simulink model "multiModeQuad_ROS"  (R2021b)
settings: Solver=FixedStepAuto  StartTime=0.0  StopTime=Inf  FixedStep=0.002  RelTol=1e-3
model workspace (MAT data in the model file):
  armLength = 0.12
  deltaT = 0.0019
  motorLength = 0.02
  servoLength = 0.03
undefined symbols (not defined in the file): AngularVelocity, Header, LinearAcceleration, Orientation, Pose
libraries: robotlib x12, slpidlib x7, sharedtransform x2, shared6dof x1
settings Model: Creator=hexia  LastModifiedBy=jack
settings OptimizationCC: EnhancedBackFolding=on  PassReuseOutputArgsAs=Individual arguments  ZeroExternalMemoryAtStartup=off  ZeroInternalMemoryAtStartup=off  MaxStackSize=64  OptimizeBlockOrder=speed  DifferentSizesBufferReuse=on  OptimizationCustomize=off  EfficientTunableParamExpr=on
settings DebuggingCC: ParameterTunabilityLossMsg=error
settings HardwareCC: ProdBitPerPointer=32  ProdBitPerSizeT=32  ProdBitPerPtrDiffT=32  ProdLargestAtomicFloat=None  ProdIntDivRoundTo=Undefined  ProdEndianess=Unspecified  ProdWordSize=32  ProdHWDeviceType=Generic->Unspecified (assume 32-bit Generic)
settings SFSimCC: MATLABDynamicMemAlloc=off
settings RTWCC: Description=Embedded Coder  SystemTargetFile=ert.tlc  HardwareBoard=Robot Operating System (ROS)  TLCOptions="-aInlineSetEventsForThisBaseRateFcn=TLC_FALSE -aSuppressMultiTaskScheduler=TLC_FALSE  -aRateBasedStepFcn=0"  TemplateMakefile=ert_default_tmf  Toolchain=Catkin  TargetLang=C++
settings CodeAppCC: ForceParamTrailComments=on  IgnoreCustomStorageClasses=off  OperatorAnnotations=on  SimulinkDataObjDesc=on  SFDataObjDesc=on  InsertBlockDesc=on
settings ERTTargetCC: SupportContinuousTime=on  SupportVariableSizeSignals=on

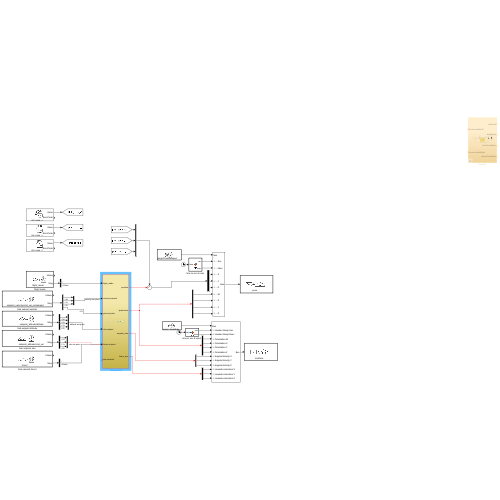
[thumbnail: Simulink's stored preview of the top-level diagram]
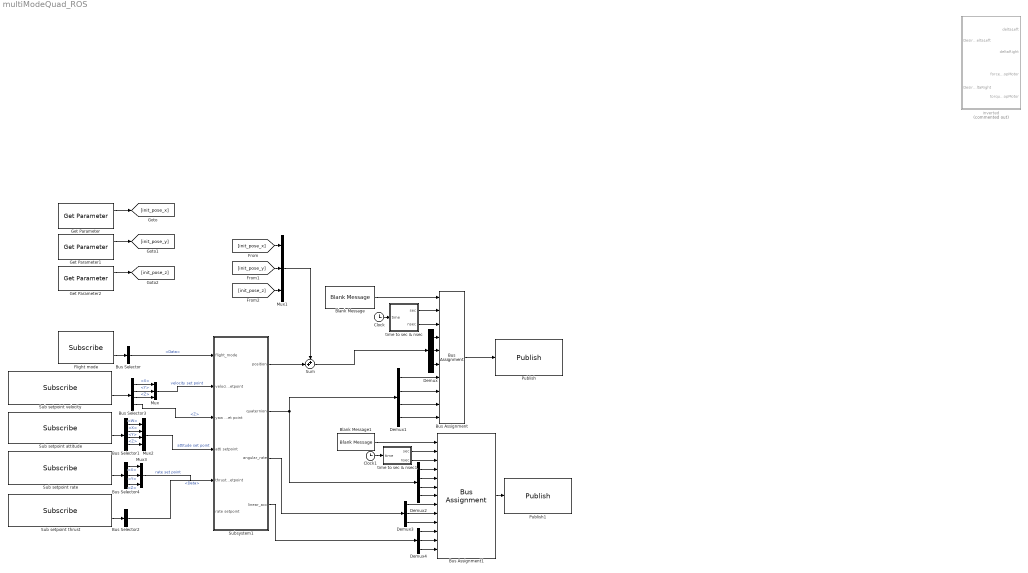
== system multiModeQuad_ROS ==
  Blank Message : robotlib/Blank Message  messageClass=Message  entityType=geometry_msgs/PoseStamped  messageType=geometry_msgs/PoseStamped  SampleTime=inf  legacyBusStruct=off
  Blank Message1 : robotlib/Blank Message  messageClass=Message  entityType=sensor_msgs/Imu  messageType=sensor_msgs/Imu  SampleTime=inf  legacyBusStruct=off
  Bus Assignment : BusAssignment  AssignedSignals=Header.Stamp.Sec,Header.Stamp.Nsec,Pose.Position.X,Pose.Position.Y,Pose.Position.Z,Pose.Orientation.W,Pose.Orientation.X,Pose.Orientation.Y,Pose.Orientation.Z
  Bus Assignment1 : BusAssignment  AssignedSignals=Header.Stamp.Sec,Header.Stamp.Nsec,Orientation.W,Orientation.X,Orientation.Y,Orientation.Z,AngularVelocity.X,AngularVelocity.Y,AngularVelocity.Z,LinearAcceleration.X,LinearAcceleration.Y,LinearAcceleration.Z
  Bus Selector : BusSelector  OutputSignals=Data
  Bus Selector1 : BusSelector  OutputSignals=Pose.Orientation.W,Pose.Orientation.X,Pose.Orientation.Y,Pose.Orientation.Z
  Bus Selector2 : BusSelector  OutputSignals=Data
  Bus Selector3 : BusSelector  OutputSignals=Linear.X,Linear.Y,Linear.Z,Angular.Z
  Bus Selector4 : BusSelector  OutputSignals=Twist.Angular.X,Twist.Angular.Y,Twist.Angular.Z
  Clock : Clock
  Clock1 : Clock
  Demux : Demux  Outputs=3
  Demux1 : Demux
  Demux2 : Demux
  Demux3 : Demux  Outputs=3
  Demux4 : Demux  Outputs=3
  Flight mode : robotlib/Subscribe  topicSource=Specify your own  topic=flight_mode  messageType=std_msgs/Int16  SampleTime=-1  legacyBusStruct=off  messageQueueLength=51
  Get Parameter : robotlib/Get Parameter  ParameterSource=Specify your own  ParameterName=init_pose_x  ParameterType=double  ParameterMaxArrayLength=16  ParameterInitialValue=0.0  SampleTime=-1  ShowErrorCodeOutput=on  ModelName=multiModeQuad_ROS  BlockId=ParamGet_multiModeQuad_ROS_459
      settings: SourceProductBaseCode=RR
  Get Parameter1 : robotlib/Get Parameter  ParameterSource=Specify your own  ParameterName=init_pose_y  ParameterType=double  ParameterMaxArrayLength=16  ParameterInitialValue=0.0  SampleTime=-1  ShowErrorCodeOutput=on  ModelName=multiModeQuad_ROS  BlockId=ParamGet_multiModeQuad_ROS_460
      settings: SourceProductBaseCode=RR
  Get Parameter2 : robotlib/Get Parameter  ParameterSource=Specify your own  ParameterName=init_pose_z  ParameterType=double  ParameterMaxArrayLength=16  ParameterInitialValue=0.0  SampleTime=-1  ShowErrorCodeOutput=on  ModelName=multiModeQuad_ROS  BlockId=ParamGet_multiModeQuad_ROS_461
      settings: SourceProductBaseCode=RR
  Mux : Mux  Inputs=3
  Mux1 : Mux  Inputs=3
  Mux2 : Mux
  Mux3 : Mux  Inputs=3
  Publish : robotlib/Publish  topicSource=Specify your own  topic=pose  messageType=geometry_msgs/PoseStamped  legacyBusStruct=off  messageQueueLength=1
  Publish1 : robotlib/Publish  topicSource=Specify your own  topic=imuData  messageType=sensor_msgs/Imu  legacyBusStruct=off  messageQueueLength=1
  Sub setpoint attitude : robotlib/Subscribe  topicSource=Specify your own  topic=setpoint_attitude/attitude  messageType=geometry_msgs/PoseStamped  SampleTime=-1  legacyBusStruct=off  messageQueueLength=51
  Sub setpoint rate : robotlib/Subscribe  topicSource=Specify your own  topic=setpoint_attitude/cmd_vel  messageType=geometry_msgs/TwistStamped  SampleTime=-1  legacyBusStruct=off  messageQueueLength=51
  Sub setpoint thrust : robotlib/Subscribe  topicSource=Specify your own  topic=thrust  messageType=std_msgs/Float32  SampleTime=-1  legacyBusStruct=off  messageQueueLength=51
  Sub setpoint velocity : robotlib/Subscribe  topicSource=Specify your own  topic=setpoint_velocity/cmd_vel_unstamped  messageType=geometry_msgs/Twist  SampleTime=-1  legacyBusStruct=off  messageQueueLength=51
  Subsystem1 : Subsystem
  Sum : Sum  Inputs=++|
  inverted : Subsystem  Commented=on
  time to sec & nsec : MATLAB Function  TreatAsAtomicUnit=on
  time to sec & nsec1 : MATLAB Function  TreatAsAtomicUnit=on
  wires:
  Mux/1 -> Subsystem1/2(velocity setpoint)  "velocity set point"
  Bus Selector3/4 -> Subsystem1/3(yaw set point)  "<Z>"
  Sub setpoint velocity/2 -> Bus Selector3/1
  Bus Selector3/3 -> Mux/3  "<Z>"
  Bus Selector3/1 -> Mux/1  "<X>"
  Bus Selector3/2 -> Mux/2  "<Y>"
  Blank Message/1 -> Bus Assignment/1
  Bus Assignment/1 -> Publish/1
  Clock/1 -> time to sec & nsec/1(time)
  time to sec & nsec/1(sec) -> Bus Assignment/2
  time to sec & nsec/2(nsec) -> Bus Assignment/3
  Demux/1 -> Bus Assignment/4
  Demux/2 -> Bus Assignment/5
  Demux/3 -> Bus Assignment/6
  Sum/1 -> Demux/1
  Demux1/1 -> Bus Assignment/7
  Demux1/2 -> Bus Assignment/8
  Demux1/3 -> Bus Assignment/9
  Demux1/4 -> Bus Assignment/10
  Get Parameter/1 -> [init_pose_x]
  Get Parameter1/1 -> [init_pose_y]
  Get Parameter2/1 -> [init_pose_z]
  Subsystem1/1(position) -> Sum/2
  Mux1/1 -> Sum/1
  [init_pose_x] -> Mux1/1
  [init_pose_y] -> Mux1/2
  [init_pose_z] -> Mux1/3
  Flight mode/2 -> Bus Selector/1
  Bus Selector/1 -> Subsystem1/1(flight_mode)  "<Data>"
  Bus Assignment1/1 -> Publish1/1
  Blank Message1/1 -> Bus Assignment1/1
  Demux2/2 -> Bus Assignment1/5
  Demux2/4 -> Bus Assignment1/7
  Demux2/1 -> Bus Assignment1/4
  Demux2/3 -> Bus Assignment1/6
  Subsystem1/2(quaternion) -> Demux1/1, Demux2/1
  Demux3/1 -> Bus Assignment1/8
  Demux3/2 -> Bus Assignment1/9
  Demux3/3 -> Bus Assignment1/10
  Subsystem1/3(angular_rate) -> Demux3/1
  Demux4/1 -> Bus Assignment1/11
  Demux4/2 -> Bus Assignment1/12
  Subsystem1/4(linear_acc) -> Demux4/1
  Demux4/3 -> Bus Assignment1/13
  Clock1/1 -> time to sec & nsec1/1(time)
  time to sec & nsec1/1(sec) -> Bus Assignment1/2
  time to sec & nsec1/2(nsec) -> Bus Assignment1/3
  Sub setpoint attitude/2 -> Bus Selector1/1
  Bus Selector1/1 -> Mux2/1  "<W>"
  Bus Selector1/2 -> Mux2/2  "<X>"
  Bus Selector1/3 -> Mux2/3  "<Y>"
  Bus Selector1/4 -> Mux2/4  "<Z>"
  Mux2/1 -> Subsystem1/4(atti setpoint)  "attitude set point"
  Sub setpoint thrust/2 -> Bus Selector2/1
  Bus Selector2/1 -> Subsystem1/5(thrust setpoint)  "<Data>"
  Sub setpoint rate/2 -> Bus Selector4/1
  Bus Selector4/1 -> Mux3/1  "<X>"
  Bus Selector4/2 -> Mux3/2  "<Y>"
  Bus Selector4/3 -> Mux3/3  "<Z>"
  Mux3/1 -> ?  "rate set point"

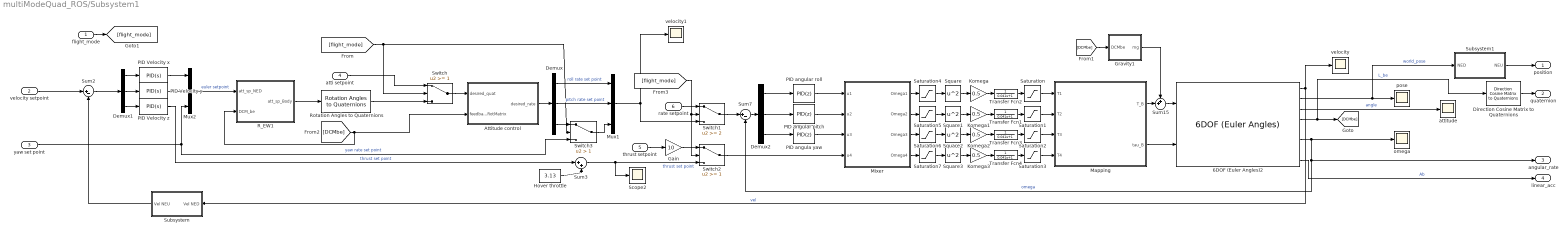
== system multiModeQuad_ROS/Subsystem1 ==
  flight_mode : Inport
  velocity setpoint : Inport  Port=2
  yaw set point : Inport  Port=3
  atti setpoint : Inport  Port=4
  thrust setpoint : Inport  Port=5
  rate setpoint : Inport  Port=6
  6DOF (Euler Angles)2 : shared6dof/6DOF (Euler Angles)  units=Metric (MKS)  mtype=Fixed  rep=Euler Angles  xme_0=[0 0 0]  Vm_0=[0 0 0]  eul_0=[0 0 0]  pm_0=[0 0 0]  mass_0=2  mass_e=0.5  mass_f=2.0  inertia=[0.015 0 0;0 0.015 0; 0 0 0.03]  inertia_e=eye(3)  inertia_f=2*eye(3)  k_quat=1.0  vre_flag=on  abi_flag=off  aMode=aMode  xme_statename=''  Vm_statename=''  eul_statename=''  quat_statename=''  pm_statename=''  mass_statename=''
      settings: SourceProductBaseCode=AE,PW,DR,MT,UV,VE
  Attitude control : MATLAB Function  TreatAsAtomicUnit=on
  Demux : Demux  Outputs=3
  Demux1 : Demux  Outputs=3
  Demux2 : Demux  Outputs=3
  Direction Cosine Matrix to Quaternions : sharedtransform/Direction Cosine Matrix  to Quaternions  aMode=0  action=None  tolerance=eps(2)
      settings: SourceProductBaseCode=AE,PW,DR,MT,UV,VE
  Gain : Gain  Gain=10
  Gravity1 : Subsystem
  Hover throttle : Constant  Value=3.13
  Komega{,1..3} (4 alike) : Gain  Gain=0.5
  Mapping : MATLAB Function  TreatAsAtomicUnit=on
  Mixer : MATLAB Function  TreatAsAtomicUnit=on
  Mux1 : Mux  Inputs=3
  Mux2 : Mux  Inputs=3
  PID Velocity x : slpidlib/PID Controller  Controller=PID  Form=Parallel  TimeDomain=Continuous-time  UseExternalTs=off  SampleTime=-1  IntegratorMethod=Forward Euler  FilterMethod=Forward Euler  ControllerParametersSource=internal  P=3  I=0  D=0.01  UseFilter=on  N=100  TunerSelectOption=Transfer Function Based (PID Tuner App)  InitialConditionSource=internal  InitialConditionForIntegrator=0  InitialConditionForFilter=0  DifferentiatorICPrevScaledInput=0  ExternalReset=none  TrackingMode=off  Kt=1  LimitOutput=off  SatLimitsSource=internal  UpperSaturationLimit=inf  LowerSaturationLimit=-inf  LinearizeAsGain=on  AntiWindupMode=none  Kb=1  POutMin=[]  POutMax=[]  IOutMin=[]  IOutMax=[]  DOutMin=[]  DOutMax=[]  NOutMin=[]  NOutMax=[]  SumOutMin=[]  SumOutMax=[]  SaturationOutMin=[]  SaturationOutMax=[]  PParamMin=[]  PParamMax=[]  IParamMin=[]  IParamMax=[]  DParamMin=[]  DParamMax=[]  NParamMin=[]  NParamMax=[]  KbParamMin=[]  KbParamMax=[]  KtParamMin=[]  KtParamMax=[]  KbOutMin=[]  KbOutMax=[]  KtOutMin=[]  KtOutMax=[]  IntegratorOutMin=[]  IntegratorOutMax=[]  FilterOutMin=[]  FilterOutMax=[]  SumI1OutMin=[]  SumI1OutMax=[]  SumI2OutMin=[]  SumI2OutMax=[]  SumI3OutMin=[]  SumI3OutMax=[]  SumI4OutMin=[]  SumI4OutMax=[]  SumDOutMin=[]  SumDOutMax=[]  DifferentiatorOutMin=[]  DifferentiatorOutMax=[]  FilterDiffOutCoefMin=[]  FilterDiffOutCoefMax=[]  ReciprocalOutMin=[]  ReciprocalOutMax=[]  SumDenOutMin=[]  SumDenOutMax=[]  SumNumOutMin=[]  SumNumOutMax=[]  DivideOutMin=[]  DivideOutMax=[]  UdiffTsProdOutMin=[]  UdiffTsProdOutMax=[]  NTsProdOutMin=[]  NTsProdOutMax=[]  UintegralTsProdOutMin=[]  UintegralTsProdOutMax=[]  UngainTsProdOutMin=[]  UngainTsProdOutMax=[]  IntegratorContinuousStateAttributes=''  IntegratorStateMustResolveToSignalObject=off  IntegratorRTWStateStorageClass=Auto  FilterContinuousStateAttributes=''  FilterStateMustResolveToSignalObject=off  FilterRTWStateStorageClass=Auto  ParallelPVariant=InternalParameters  IdealPVariant=Disabled  IVariant=InternalParameters  DVariant=InternalParameters  IntegratorVariant=Continuous  SatVariant=Disabled  AWVariant=Passthrough  PCopyVariant=Disabled  TRVariant=Disabled  FdbkBlocksVariant=Forward  IdealPFdbkVariant=Disabled  SatFdbkVariant=Disabled  DerivativeFilterVariant=ContFilter  NVariant=InternalParameters  NCopyVariant=Disabled  FilterICVariant=InternalICsFilter  IntegratorICVariant=InternalICs  ExternalResetVariant=Disabled  TRSumVariant=Passthrough  SumFdbkVariant=Disabled  SumVariant=Sum_PID  TsampFilterVariant=InternalTs  TsampNgainVariant=Passthrough  TsampIntegralVariant=Passthrough  ExternalSaturationOutDataTypeStr=Inherit: Same as second input
  PID Velocity y : slpidlib/PID Controller  Controller=PID  Form=Parallel  TimeDomain=Continuous-time  UseExternalTs=off  SampleTime=-1  IntegratorMethod=Forward Euler  FilterMethod=Forward Euler  ControllerParametersSource=internal  P=3  I=0.02  D=0.01  UseFilter=on  N=100  TunerSelectOption=Transfer Function Based (PID Tuner App)  InitialConditionSource=internal  InitialConditionForIntegrator=0  InitialConditionForFilter=0  DifferentiatorICPrevScaledInput=0  ExternalReset=none  TrackingMode=off  Kt=1  LimitOutput=off  SatLimitsSource=internal  UpperSaturationLimit=inf  LowerSaturationLimit=-inf  LinearizeAsGain=on  AntiWindupMode=none  Kb=1  POutMin=[]  POutMax=[]  IOutMin=[]  IOutMax=[]  DOutMin=[]  DOutMax=[]  NOutMin=[]  NOutMax=[]  SumOutMin=[]  SumOutMax=[]  SaturationOutMin=[]  SaturationOutMax=[]  PParamMin=[]  PParamMax=[]  IParamMin=[]  IParamMax=[]  DParamMin=[]  DParamMax=[]  NParamMin=[]  NParamMax=[]  KbParamMin=[]  KbParamMax=[]  KtParamMin=[]  KtParamMax=[]  KbOutMin=[]  KbOutMax=[]  KtOutMin=[]  KtOutMax=[]  IntegratorOutMin=[]  IntegratorOutMax=[]  FilterOutMin=[]  FilterOutMax=[]  SumI1OutMin=[]  SumI1OutMax=[]  SumI2OutMin=[]  SumI2OutMax=[]  SumI3OutMin=[]  SumI3OutMax=[]  SumI4OutMin=[]  SumI4OutMax=[]  SumDOutMin=[]  SumDOutMax=[]  DifferentiatorOutMin=[]  DifferentiatorOutMax=[]  FilterDiffOutCoefMin=[]  FilterDiffOutCoefMax=[]  ReciprocalOutMin=[]  ReciprocalOutMax=[]  SumDenOutMin=[]  SumDenOutMax=[]  SumNumOutMin=[]  SumNumOutMax=[]  DivideOutMin=[]  DivideOutMax=[]  UdiffTsProdOutMin=[]  UdiffTsProdOutMax=[]  NTsProdOutMin=[]  NTsProdOutMax=[]  UintegralTsProdOutMin=[]  UintegralTsProdOutMax=[]  UngainTsProdOutMin=[]  UngainTsProdOutMax=[]  IntegratorContinuousStateAttributes=''  IntegratorStateMustResolveToSignalObject=off  IntegratorRTWStateStorageClass=Auto  FilterContinuousStateAttributes=''  FilterStateMustResolveToSignalObject=off  FilterRTWStateStorageClass=Auto  ParallelPVariant=InternalParameters  IdealPVariant=Disabled  IVariant=InternalParameters  DVariant=InternalParameters  IntegratorVariant=Continuous  SatVariant=Disabled  AWVariant=Passthrough  PCopyVariant=Disabled  TRVariant=Disabled  FdbkBlocksVariant=Forward  IdealPFdbkVariant=Disabled  SatFdbkVariant=Disabled  DerivativeFilterVariant=ContFilter  NVariant=InternalParameters  NCopyVariant=Disabled  FilterICVariant=InternalICsFilter  IntegratorICVariant=InternalICs  ExternalResetVariant=Disabled  TRSumVariant=Passthrough  SumFdbkVariant=Disabled  SumVariant=Sum_PID  TsampFilterVariant=InternalTs  TsampNgainVariant=Passthrough  TsampIntegralVariant=Passthrough  ExternalSaturationOutDataTypeStr=Inherit: Same as second input
  PID Velocity z : slpidlib/PID Controller  Controller=PID  Form=Parallel  TimeDomain=Continuous-time  UseExternalTs=off  SampleTime=-1  IntegratorMethod=Forward Euler  FilterMethod=Forward Euler  ControllerParametersSource=internal  P=3  I=0.2  D=2  UseFilter=on  N=100  TunerSelectOption=Transfer Function Based (PID Tuner App)  InitialConditionSource=internal  InitialConditionForIntegrator=0  InitialConditionForFilter=0  DifferentiatorICPrevScaledInput=0  ExternalReset=none  TrackingMode=off  Kt=1  LimitOutput=off  SatLimitsSource=internal  UpperSaturationLimit=inf  LowerSaturationLimit=-inf  LinearizeAsGain=on  AntiWindupMode=none  Kb=1  POutMin=[]  POutMax=[]  IOutMin=[]  IOutMax=[]  DOutMin=[]  DOutMax=[]  NOutMin=[]  NOutMax=[]  SumOutMin=[]  SumOutMax=[]  SaturationOutMin=[]  SaturationOutMax=[]  PParamMin=[]  PParamMax=[]  IParamMin=[]  IParamMax=[]  DParamMin=[]  DParamMax=[]  NParamMin=[]  NParamMax=[]  KbParamMin=[]  KbParamMax=[]  KtParamMin=[]  KtParamMax=[]  KbOutMin=[]  KbOutMax=[]  KtOutMin=[]  KtOutMax=[]  IntegratorOutMin=[]  IntegratorOutMax=[]  FilterOutMin=[]  FilterOutMax=[]  SumI1OutMin=[]  SumI1OutMax=[]  SumI2OutMin=[]  SumI2OutMax=[]  SumI3OutMin=[]  SumI3OutMax=[]  SumI4OutMin=[]  SumI4OutMax=[]  SumDOutMin=[]  SumDOutMax=[]  DifferentiatorOutMin=[]  DifferentiatorOutMax=[]  FilterDiffOutCoefMin=[]  FilterDiffOutCoefMax=[]  ReciprocalOutMin=[]  ReciprocalOutMax=[]  SumDenOutMin=[]  SumDenOutMax=[]  SumNumOutMin=[]  SumNumOutMax=[]  DivideOutMin=[]  DivideOutMax=[]  UdiffTsProdOutMin=[]  UdiffTsProdOutMax=[]  NTsProdOutMin=[]  NTsProdOutMax=[]  UintegralTsProdOutMin=[]  UintegralTsProdOutMax=[]  UngainTsProdOutMin=[]  UngainTsProdOutMax=[]  IntegratorContinuousStateAttributes=''  IntegratorStateMustResolveToSignalObject=off  IntegratorRTWStateStorageClass=Auto  FilterContinuousStateAttributes=''  FilterStateMustResolveToSignalObject=off  FilterRTWStateStorageClass=Auto  ParallelPVariant=InternalParameters  IdealPVariant=Disabled  IVariant=InternalParameters  DVariant=InternalParameters  IntegratorVariant=Continuous  SatVariant=Disabled  AWVariant=Passthrough  PCopyVariant=Disabled  TRVariant=Disabled  FdbkBlocksVariant=Forward  IdealPFdbkVariant=Disabled  SatFdbkVariant=Disabled  DerivativeFilterVariant=ContFilter  NVariant=InternalParameters  NCopyVariant=Disabled  FilterICVariant=InternalICsFilter  IntegratorICVariant=InternalICs  ExternalResetVariant=Disabled  TRSumVariant=Passthrough  SumFdbkVariant=Disabled  SumVariant=Sum_PID  TsampFilterVariant=InternalTs  TsampNgainVariant=Passthrough  TsampIntegralVariant=Passthrough  ExternalSaturationOutDataTypeStr=Inherit: Same as second input
  PID angula yaw : slpidlib/PID Controller  Controller=PID  Form=Ideal  TimeDomain=Discrete-time  UseExternalTs=off  SampleTime=-1  IntegratorMethod=Forward Euler  FilterMethod=Forward Euler  ControllerParametersSource=internal  P=1  I=0.05  D=0.04  UseFilter=on  N=300  TunerSelectOption=Transfer Function Based (PID Tuner App)  InitialConditionSource=internal  InitialConditionForIntegrator=0  InitialConditionForFilter=0  DifferentiatorICPrevScaledInput=0  ExternalReset=none  TrackingMode=off  Kt=1  LimitOutput=off  SatLimitsSource=internal  UpperSaturationLimit=inf  LowerSaturationLimit=-inf  LinearizeAsGain=on  AntiWindupMode=none  Kb=1  POutMin=[]  POutMax=[]  IOutMin=[]  IOutMax=[]  DOutMin=[]  DOutMax=[]  NOutMin=[]  NOutMax=[]  SumOutMin=[]  SumOutMax=[]  SaturationOutMin=[]  SaturationOutMax=[]  PParamMin=[]  PParamMax=[]  IParamMin=[]  IParamMax=[]  DParamMin=[]  DParamMax=[]  NParamMin=[]  NParamMax=[]  KbParamMin=[]  KbParamMax=[]  KtParamMin=[]  KtParamMax=[]  KbOutMin=[]  KbOutMax=[]  KtOutMin=[]  KtOutMax=[]  IntegratorOutMin=[]  IntegratorOutMax=[]  FilterOutMin=[]  FilterOutMax=[]  SumI1OutMin=[]  SumI1OutMax=[]  SumI2OutMin=[]  SumI2OutMax=[]  SumI3OutMin=[]  SumI3OutMax=[]  SumI4OutMin=[]  SumI4OutMax=[]  SumDOutMin=[]  SumDOutMax=[]  DifferentiatorOutMin=[]  DifferentiatorOutMax=[]  FilterDiffOutCoefMin=[]  FilterDiffOutCoefMax=[]  ReciprocalOutMin=[]  ReciprocalOutMax=[]  SumDenOutMin=[]  SumDenOutMax=[]  SumNumOutMin=[]  SumNumOutMax=[]  DivideOutMin=[]  DivideOutMax=[]  UdiffTsProdOutMin=[]  UdiffTsProdOutMax=[]  NTsProdOutMin=[]  NTsProdOutMax=[]  UintegralTsProdOutMin=[]  UintegralTsProdOutMax=[]  UngainTsProdOutMin=[]  UngainTsProdOutMax=[]  IntegratorContinuousStateAttributes=''  IntegratorStateMustResolveToSignalObject=off  IntegratorRTWStateStorageClass=Auto  FilterContinuousStateAttributes=''  FilterStateMustResolveToSignalObject=off  FilterRTWStateStorageClass=Auto  ParallelPVariant=Passthrough  IdealPVariant=InternalParameters  IVariant=InternalParameters  DVariant=InternalParameters  IntegratorVariant=Discrete  SatVariant=Disabled  AWVariant=Passthrough  PCopyVariant=Disabled  TRVariant=Disabled  FdbkBlocksVariant=Forward  IdealPFdbkVariant=Disabled  SatFdbkVariant=Disabled  DerivativeFilterVariant=ForwardEulerFilter  NVariant=InternalParameters  NCopyVariant=Disabled  FilterICVariant=InternalICsFilter  IntegratorICVariant=InternalICs  ExternalResetVariant=Disabled  TRSumVariant=Passthrough  SumFdbkVariant=Disabled  SumVariant=Sum_PID  TsampFilterVariant=InternalTs  TsampNgainVariant=Passthrough  TsampIntegralVariant=Passthrough  ExternalSaturationOutDataTypeStr=Inherit: Same as second input
  PID angular pitch : slpidlib/PID Controller  Controller=PID  Form=Ideal  TimeDomain=Discrete-time  UseExternalTs=off  SampleTime=-1  IntegratorMethod=Forward Euler  FilterMethod=Forward Euler  ControllerParametersSource=internal  P=0.6  I=0.05  D=0.05  UseFilter=on  N=300  TunerSelectOption=Transfer Function Based (PID Tuner App)  InitialConditionSource=internal  InitialConditionForIntegrator=0  InitialConditionForFilter=0  DifferentiatorICPrevScaledInput=0  ExternalReset=none  TrackingMode=off  Kt=1  LimitOutput=off  SatLimitsSource=internal  UpperSaturationLimit=inf  LowerSaturationLimit=-inf  LinearizeAsGain=on  AntiWindupMode=none  Kb=1  POutMin=[]  POutMax=[]  IOutMin=[]  IOutMax=[]  DOutMin=[]  DOutMax=[]  NOutMin=[]  NOutMax=[]  SumOutMin=[]  SumOutMax=[]  SaturationOutMin=[]  SaturationOutMax=[]  PParamMin=[]  PParamMax=[]  IParamMin=[]  IParamMax=[]  DParamMin=[]  DParamMax=[]  NParamMin=[]  NParamMax=[]  KbParamMin=[]  KbParamMax=[]  KtParamMin=[]  KtParamMax=[]  KbOutMin=[]  KbOutMax=[]  KtOutMin=[]  KtOutMax=[]  IntegratorOutMin=[]  IntegratorOutMax=[]  FilterOutMin=[]  FilterOutMax=[]  SumI1OutMin=[]  SumI1OutMax=[]  SumI2OutMin=[]  SumI2OutMax=[]  SumI3OutMin=[]  SumI3OutMax=[]  SumI4OutMin=[]  SumI4OutMax=[]  SumDOutMin=[]  SumDOutMax=[]  DifferentiatorOutMin=[]  DifferentiatorOutMax=[]  FilterDiffOutCoefMin=[]  FilterDiffOutCoefMax=[]  ReciprocalOutMin=[]  ReciprocalOutMax=[]  SumDenOutMin=[]  SumDenOutMax=[]  SumNumOutMin=[]  SumNumOutMax=[]  DivideOutMin=[]  DivideOutMax=[]  UdiffTsProdOutMin=[]  UdiffTsProdOutMax=[]  NTsProdOutMin=[]  NTsProdOutMax=[]  UintegralTsProdOutMin=[]  UintegralTsProdOutMax=[]  UngainTsProdOutMin=[]  UngainTsProdOutMax=[]  IntegratorContinuousStateAttributes=''  IntegratorStateMustResolveToSignalObject=off  IntegratorRTWStateStorageClass=Auto  FilterContinuousStateAttributes=''  FilterStateMustResolveToSignalObject=off  FilterRTWStateStorageClass=Auto  ParallelPVariant=Passthrough  IdealPVariant=InternalParameters  IVariant=InternalParameters  DVariant=InternalParameters  IntegratorVariant=Discrete  SatVariant=Disabled  AWVariant=Passthrough  PCopyVariant=Disabled  TRVariant=Disabled  FdbkBlocksVariant=Forward  IdealPFdbkVariant=Disabled  SatFdbkVariant=Disabled  DerivativeFilterVariant=ForwardEulerFilter  NVariant=InternalParameters  NCopyVariant=Disabled  FilterICVariant=InternalICsFilter  IntegratorICVariant=InternalICs  ExternalResetVariant=Disabled  TRSumVariant=Passthrough  SumFdbkVariant=Disabled  SumVariant=Sum_PID  TsampFilterVariant=InternalTs  TsampNgainVariant=Passthrough  TsampIntegralVariant=Passthrough  ExternalSaturationOutDataTypeStr=Inherit: Same as second input
  PID angular roll : slpidlib/PID Controller  Controller=PID  Form=Ideal  TimeDomain=Discrete-time  UseExternalTs=off  SampleTime=-1  IntegratorMethod=Forward Euler  FilterMethod=Forward Euler  ControllerParametersSource=internal  P=0.6  I=0.05  D=0.05  UseFilter=on  N=300  TunerSelectOption=Transfer Function Based (PID Tuner App)  InitialConditionSource=internal  InitialConditionForIntegrator=0  InitialConditionForFilter=0  DifferentiatorICPrevScaledInput=0  ExternalReset=none  TrackingMode=off  Kt=1  LimitOutput=off  SatLimitsSource=internal  UpperSaturationLimit=inf  LowerSaturationLimit=-inf  LinearizeAsGain=on  AntiWindupMode=none  Kb=1  POutMin=[]  POutMax=[]  IOutMin=[]  IOutMax=[]  DOutMin=[]  DOutMax=[]  NOutMin=[]  NOutMax=[]  SumOutMin=[]  SumOutMax=[]  SaturationOutMin=[]  SaturationOutMax=[]  PParamMin=[]  PParamMax=[]  IParamMin=[]  IParamMax=[]  DParamMin=[]  DParamMax=[]  NParamMin=[]  NParamMax=[]  KbParamMin=[]  KbParamMax=[]  KtParamMin=[]  KtParamMax=[]  KbOutMin=[]  KbOutMax=[]  KtOutMin=[]  KtOutMax=[]  IntegratorOutMin=[]  IntegratorOutMax=[]  FilterOutMin=[]  FilterOutMax=[]  SumI1OutMin=[]  SumI1OutMax=[]  SumI2OutMin=[]  SumI2OutMax=[]  SumI3OutMin=[]  SumI3OutMax=[]  SumI4OutMin=[]  SumI4OutMax=[]  SumDOutMin=[]  SumDOutMax=[]  DifferentiatorOutMin=[]  DifferentiatorOutMax=[]  FilterDiffOutCoefMin=[]  FilterDiffOutCoefMax=[]  ReciprocalOutMin=[]  ReciprocalOutMax=[]  SumDenOutMin=[]  SumDenOutMax=[]  SumNumOutMin=[]  SumNumOutMax=[]  DivideOutMin=[]  DivideOutMax=[]  UdiffTsProdOutMin=[]  UdiffTsProdOutMax=[]  NTsProdOutMin=[]  NTsProdOutMax=[]  UintegralTsProdOutMin=[]  UintegralTsProdOutMax=[]  UngainTsProdOutMin=[]  UngainTsProdOutMax=[]  IntegratorContinuousStateAttributes=''  IntegratorStateMustResolveToSignalObject=off  IntegratorRTWStateStorageClass=Auto  FilterContinuousStateAttributes=''  FilterStateMustResolveToSignalObject=off  FilterRTWStateStorageClass=Auto  ParallelPVariant=Passthrough  IdealPVariant=InternalParameters  IVariant=InternalParameters  DVariant=InternalParameters  IntegratorVariant=Discrete  SatVariant=Disabled  AWVariant=Passthrough  PCopyVariant=Disabled  TRVariant=Disabled  FdbkBlocksVariant=Forward  IdealPFdbkVariant=Disabled  SatFdbkVariant=Disabled  DerivativeFilterVariant=ForwardEulerFilter  NVariant=InternalParameters  NCopyVariant=Disabled  FilterICVariant=InternalICsFilter  IntegratorICVariant=InternalICs  ExternalResetVariant=Disabled  TRSumVariant=Passthrough  SumFdbkVariant=Disabled  SumVariant=Sum_PID  TsampFilterVariant=InternalTs  TsampNgainVariant=Passthrough  TsampIntegralVariant=Passthrough  ExternalSaturationOutDataTypeStr=Inherit: Same as second input
  R_EW1 : MATLAB Function  TreatAsAtomicUnit=on
  Rotation Angles to Quaternions : sharedtransform/Rotation Angles to Quaternions  rotationOrder=ZYX  aMode=aMode
      settings: SourceProductBaseCode=AE,PW,DR,MT,UV,VE
  Saturation{,1..3} (4 alike) : Saturate  UpperLimit=10  LowerLimit=0
  Saturation{4..7} (4 alike) : Saturate  UpperLimit=inf  LowerLimit=0
  Scope2 : Scope
  Square{,1..3} (4 alike) : Math  Operator=square  SaturateOnIntegerOverflow=on
  Subsystem : Subsystem
  Subsystem1 : Subsystem
  Sum15 : Sum  Inputs=++|
  Sum2 : Sum  Inputs=|+-
  Sum3 : Sum  Inputs=|++
  Sum7 : Sum  Inputs=|+-
  Switch : Switch  Threshold=1
  Switch1 : Switch  Threshold=2
  Switch2 : Switch  Threshold=1
  Switch3 : Switch  Criteria=u2 > Threshold  Threshold=1
  Transfer Fcn{1..4} (4 alike) : TransferFcn  Denominator=[0.041 1]
  attitude : Scope
  omega : Scope
  pose : Scope
  velocity : Scope
  velocity1 : Scope
  position : Outport
  quaternion : Outport  Port=2
  angular_rate : Outport  Port=3
  linear_acc : Outport  Port=4
  wires:
  6DOF (Euler Angles)2/3 -> attitude/1  "angle"
  6DOF (Euler Angles)2/2 -> Subsystem1/1(NED), pose/1  "world_pose"
  Switch1/1 -> Sum7/1
  Demux1/3 -> PID Velocity z/1
  Mixer/1(Omega1) -> Saturation4/1
  Attitude control/1(desired_rate) -> Demux/1
  6DOF (Euler Angles)2/6 -> Sum7/2, angular_rate/1, omega/1  "omega"
  Saturation4/1 -> Square/1
  Mixer/2(Omega2) -> Saturation5/1
  PID angular pitch/1 -> Mixer/2(u2)
  Saturation6/1 -> Square2/1
  Sum7/1 -> Demux2/1
  Sum15/1 -> 6DOF (Euler Angles)2/1
  Transfer Fcn2/1 -> Saturation/1
  Mixer/3(Omega3) -> Saturation6/1
  Hover throttle/1 -> Sum3/2
  PID angular roll/1 -> Mixer/1(u1)
  Mapping/2(tau_B) -> 6DOF (Euler Angles)2/2
  6DOF (Euler Angles)2/4 -> Direction Cosine Matrix to Quaternions/1, [DCMbe]  "L_be"
  Komega2/1 -> Transfer Fcn3/1
  PID angula yaw/1 -> Mixer/3(u3)
  PID Velocity z/1 -> Sum3/1  "thrust set point"
  6DOF (Euler Angles)2/1 -> velocity/1, Subsystem/1(Vel NED)  "vel"
  PID Velocity x/1 -> Mux2/1
  Gravity1/1(mg) -> Sum15/1
  Saturation5/1 -> Square1/1
  Demux2/3 -> PID angula yaw/1
  Mux2/1 -> R_EW1/1(att_sp_NED)  "euler setpoint"
  Demux2/2 -> PID angular pitch/1
  Demux/1 -> Mux1/1  "roll rate set point"
  Transfer Fcn3/1 -> Saturation2/1
  Demux1/2 -> PID Velocity y/1
  Mapping/1(T_B) -> Sum15/2
  Komega/1 -> Transfer Fcn2/1
  Square3/1 -> Komega3/1
  Saturation3/1 -> Mapping/4(T4)
  Saturation1/1 -> Mapping/2(T2)
  Transfer Fcn4/1 -> Saturation3/1
  Saturation2/1 -> Mapping/3(T3)
  Square/1 -> Komega/1
  Transfer Fcn1/1 -> Saturation1/1
  Sum3/1 -> Scope2/1, Switch2/3  "thrust set point"
  Komega3/1 -> Transfer Fcn4/1
  Demux2/1 -> PID angular roll/1
  Demux1/1 -> PID Velocity x/1
  Square1/1 -> Komega1/1
  Mixer/4(Omega4) -> Saturation7/1
  [DCMbe] -> R_EW1/2(DCM_be), Attitude control/2(feedback_RotMatrix)
  Saturation7/1 -> Square3/1
  PID Velocity y/1 -> Mux2/2
  velocity setpoint/1 -> Sum2/1
  Subsystem/1(Vel NEU) -> Sum2/2
  Komega1/1 -> Transfer Fcn1/1
  Saturation/1 -> Mapping/1(T1)
  Square2/1 -> Komega2/1
  Sum2/1 -> Demux1/1
  [DCMbe] -> Gravity1/1(DCMbe)
  Demux/2 -> Mux1/2  "pitch rate set point"
  yaw set point/1 -> Switch3/3, Mux2/3  "yaw rate set point"
  Direction Cosine Matrix to Quaternions/1 -> quaternion/1
  Subsystem1/1(NEU) -> position/1
  6DOF (Euler Angles)2/8 -> linear_acc/1  "Ab"
  flight_mode/1 -> [flight_mode]
  Switch/1 -> Attitude control/1(desired_quat)
  atti setpoint/1 -> Switch/1
  [flight_mode] -> Switch3/2, Switch/2
  thrust setpoint/1 -> Gain/1
  Switch2/1 -> Mixer/4(u4)
  Gain/1 -> Switch2/1
  Rotation Angles to Quaternions/1 -> Switch/3
  Mux1/1 -> Switch1/3, velocity1/1
  rate setpoint/1 -> Switch1/1
  [flight_mode] -> Switch2/2, Switch1/2
  R_EW1/1(att_sp_Body) -> Rotation Angles to Quaternions/1
  Demux/3 -> Switch3/1
  Switch3/1 -> Mux1/3

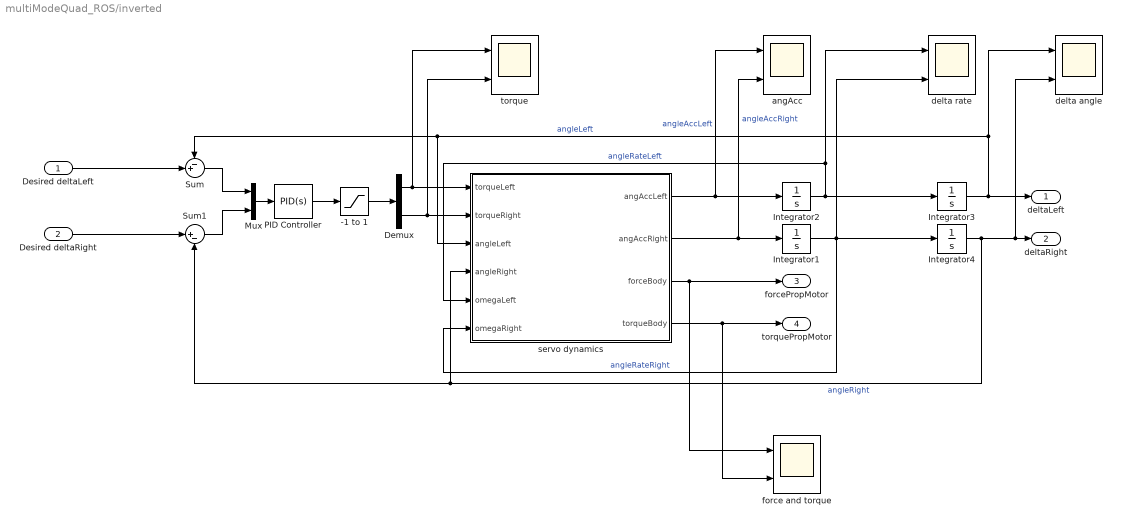
== system multiModeQuad_ROS/inverted ==
  Desired deltaLeft : Inport
  Desired deltaRight : Inport  Port=2
  -1 to 1 : Saturate  UpperLimit=0.08  LowerLimit=-0.08
  Demux : Demux  Outputs=2
  Integrator1 : Integrator  LimitOutput=on  UpperSaturationLimit=5.5  LowerSaturationLimit=-5.5
  Integrator2 : Integrator  LimitOutput=on  UpperSaturationLimit=5.5  LowerSaturationLimit=-5.5
  Integrator3 : Integrator  LimitOutput=on  UpperSaturationLimit=pi/2  LowerSaturationLimit=-pi/2
  Integrator4 : Integrator  LimitOutput=on  UpperSaturationLimit=pi/2  LowerSaturationLimit=-pi/2
  Mux : Mux  Inputs=2
  PID Controller : slpidlib/PID Controller  Controller=PID  Form=Parallel  TimeDomain=Continuous-time  UseExternalTs=off  SampleTime=-1  IntegratorMethod=Forward Euler  FilterMethod=Forward Euler  ControllerParametersSource=internal  P=0.8  I=0  D=0.022  UseFilter=on  N=500  TunerSelectOption=Transfer Function Based (PID Tuner App)  InitialConditionSource=internal  InitialConditionForIntegrator=0  InitialConditionForFilter=0  DifferentiatorICPrevScaledInput=0  ExternalReset=none  TrackingMode=off  Kt=1  LimitOutput=off  SatLimitsSource=internal  UpperSaturationLimit=inf  LowerSaturationLimit=-inf  LinearizeAsGain=on  AntiWindupMode=none  Kb=1  POutMin=[]  POutMax=[]  IOutMin=[]  IOutMax=[]  DOutMin=[]  DOutMax=[]  NOutMin=[]  NOutMax=[]  SumOutMin=[]  SumOutMax=[]  SaturationOutMin=[]  SaturationOutMax=[]  PParamMin=[]  PParamMax=[]  IParamMin=[]  IParamMax=[]  DParamMin=[]  DParamMax=[]  NParamMin=[]  NParamMax=[]  KbParamMin=[]  KbParamMax=[]  KtParamMin=[]  KtParamMax=[]  KbOutMin=[]  KbOutMax=[]  KtOutMin=[]  KtOutMax=[]  IntegratorOutMin=[]  IntegratorOutMax=[]  FilterOutMin=[]  FilterOutMax=[]  SumI1OutMin=[]  SumI1OutMax=[]  SumI2OutMin=[]  SumI2OutMax=[]  SumI3OutMin=[]  SumI3OutMax=[]  SumI4OutMin=[]  SumI4OutMax=[]  SumDOutMin=[]  SumDOutMax=[]  DifferentiatorOutMin=[]  DifferentiatorOutMax=[]  FilterDiffOutCoefMin=[]  FilterDiffOutCoefMax=[]  ReciprocalOutMin=[]  ReciprocalOutMax=[]  SumDenOutMin=[]  SumDenOutMax=[]  SumNumOutMin=[]  SumNumOutMax=[]  DivideOutMin=[]  DivideOutMax=[]  UdiffTsProdOutMin=[]  UdiffTsProdOutMax=[]  NTsProdOutMin=[]  NTsProdOutMax=[]  UintegralTsProdOutMin=[]  UintegralTsProdOutMax=[]  UngainTsProdOutMin=[]  UngainTsProdOutMax=[]  IntegratorContinuousStateAttributes=''  IntegratorStateMustResolveToSignalObject=off  IntegratorRTWStateStorageClass=Auto  FilterContinuousStateAttributes=''  FilterStateMustResolveToSignalObject=off  FilterRTWStateStorageClass=Auto  ParallelPVariant=InternalParameters  IdealPVariant=Disabled  IVariant=InternalParameters  DVariant=InternalParameters  IntegratorVariant=Continuous  SatVariant=Disabled  AWVariant=Passthrough  PCopyVariant=Disabled  TRVariant=Disabled  FdbkBlocksVariant=Forward  IdealPFdbkVariant=Disabled  SatFdbkVariant=Disabled  DerivativeFilterVariant=ContFilter  NVariant=InternalParameters  NCopyVariant=Disabled  FilterICVariant=InternalICsFilter  IntegratorICVariant=InternalICs  ExternalResetVariant=Disabled  TRSumVariant=Passthrough  SumFdbkVariant=Disabled  SumVariant=Sum_PID  TsampFilterVariant=InternalTs  TsampNgainVariant=Passthrough  TsampIntegralVariant=Passthrough  ExternalSaturationOutDataTypeStr=Inherit: Same as second input
  Sum : Sum  Inputs=-+|
  Sum1 : Sum  Inputs=|+-
  angAcc : Scope  NumInputPorts=2
  delta angle : Scope  NumInputPorts=2
  delta rate : Scope  NumInputPorts=2
  force and torque : Scope  NumInputPorts=2
  servo dynamics : MATLAB Function  TreatAsAtomicUnit=on
  torque : Scope  NumInputPorts=2
  deltaLeft : Outport
  deltaRight : Outport  Port=2
  forcePropMotor : Outport  Port=3
  torquePropMotor : Outport  Port=4
  wires:
  Sum1/1 -> Mux/2
  Demux/2 -> torque/2, servo dynamics/2(torqueRight)
  servo dynamics/1(angAccLeft) -> angAcc/1, Integrator2/1  "angleAccLeft"
  servo dynamics/2(angAccRight) -> angAcc/2, Integrator1/1  "angleAccRight"
  Integrator2/1 -> servo dynamics/5(omegaLeft), delta rate/1, Integrator3/1  "angleRateLeft"
  Integrator1/1 -> servo dynamics/6(omegaRight), delta rate/2, Integrator4/1  "angleRateRight"
  Integrator3/1 -> delta angle/1, servo dynamics/3(angleLeft), Sum/1, deltaLeft/1  "angleLeft"
  Integrator4/1 -> delta angle/2, deltaRight/1, servo dynamics/4(angleRight), Sum1/2  "angleRight"
  Mux/1 -> PID Controller/1
  Sum/1 -> Mux/1
  Demux/1 -> torque/1, servo dynamics/1(torqueLeft)
  PID Controller/1 -> -1 to 1/1
  -1 to 1/1 -> Demux/1
  servo dynamics/3(forceBody) -> force and torque/1, forcePropMotor/1
  servo dynamics/4(torqueBody) -> force and torque/2, torquePropMotor/1
  Desired deltaLeft/1 -> Sum/2
  Desired deltaRight/1 -> Sum1/1

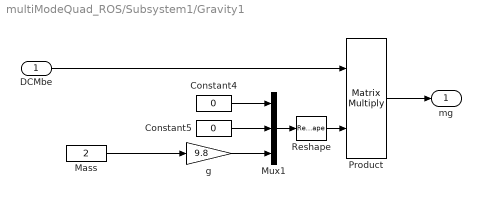
== system multiModeQuad_ROS/Subsystem1/Gravity1 ==
  DCMbe : Inport
  Constant4 : Constant  Value=0
  Constant5 : Constant  Value=0
  Mass : Constant  Value=2
  Mux1 : Mux  Inputs=3
  Product : Product  Multiplication=Matrix(*)  RndMeth=Zero
  Reshape : Reshape  OutputDimensionality=Column vector (2-D)
  g : Gain  Gain=9.8
  mg : Outport  VectorParamsAs1DForOutWhenUnconnected=off
  wires:
  Reshape/1 -> Product/2
  Product/1 -> mg/1
  Mass/1 -> g/1
  Mux1/1 -> Reshape/1
  Constant5/1 -> Mux1/2
  g/1 -> Mux1/3
  Constant4/1 -> Mux1/1
  DCMbe/1 -> Product/1

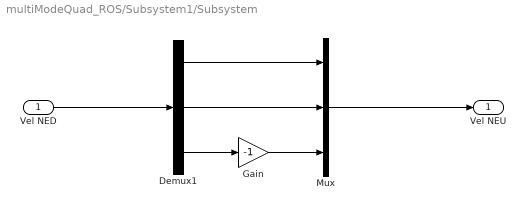
== system multiModeQuad_ROS/Subsystem1/Subsystem ==
  Vel NED : Inport
  Demux1 : Demux  Outputs=3
  Gain : Gain  Gain=-1
  Mux : Mux  Inputs=3
  Vel NEU : Outport
  wires:
  Gain/1 -> Mux/3
  Demux1/3 -> Gain/1
  Demux1/2 -> Mux/2
  Demux1/1 -> Mux/1
  Mux/1 -> Vel NEU/1
  Vel NED/1 -> Demux1/1

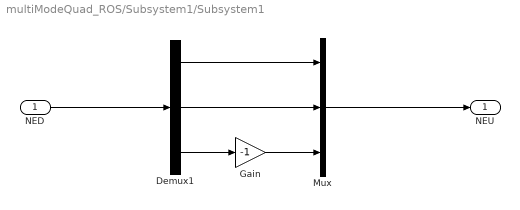
== system multiModeQuad_ROS/Subsystem1/Subsystem1 ==
  NED : Inport
  Demux1 : Demux  Outputs=3
  Gain : Gain  Gain=-1
  Mux : Mux  Inputs=3
  NEU : Outport
  wires:
  Gain/1 -> Mux/3
  Demux1/3 -> Gain/1
  Demux1/2 -> Mux/2
  Demux1/1 -> Mux/1
  Mux/1 -> NEU/1
  NED/1 -> Demux1/1

== matlab function multiModeQuad_ROS/time to sec & nsec ==
  data: time input; sec output; nsec output
function [sec, nsec] = fcn(time)
sec = floor(time);
nsec = (time - sec)*1e9;

== matlab function multiModeQuad_ROS/Subsystem1/Mixer ==
  data: Omega1 output; u1 input; Omega2 output; Omega3 output; u2 input; u3 input; u4 input; Omega4 output
%% Date created: 08/01/2020
%% Author: Jack He
%% Input remap
function [Omega1, Omega2, Omega3, Omega4] = fcn(u1,u2,u3,u4)
Omega1 = u4 - u1 - u2 - u3;
Omega2 = u4 - u1 + u2 + u3;
Omega3 = u4 + u1 - u2 + u3;
Omega4 = u4 + u1 + u2 - u3;

== matlab function multiModeQuad_ROS/Subsystem1/Attitude control ==
  data: desired_quat input; desired_rate output; feedback_RotMatrix input
function desired_rate  = fcn(desired_quat, feedback_RotMatrix)
feedback_quat = rotm2quat(feedback_RotMatrix');
quat_diff = quatmultiply(quatinv(feedback_quat), desired_quat');
axang = quat2axang(quat_diff);
desired_angle = axang(4);
desired_axis = axang(1:3)';
% desired_rate = axang(1:3)'*sign(axang(4))*0.01;
desired_rate = axang(1:3)'*axang(4);

== matlab function multiModeQuad_ROS/time to sec & nsec1 ==
  data: time input; sec output; nsec output
function [sec, nsec] = fcn(time)
sec = floor(time);
nsec = (time - sec)*1e9;

== matlab function multiModeQuad_ROS/inverted/servo dynamics ==
  data: torqueLeft input; torqueRight input; angAccLeft output; angAccRight output; angleLeft input; angleRight input; omegaLeft input; omegaRight input; forceBody output; torqueBody output; armLength parameter; servoLength parameter; motorLength parameter
%% Date crreated: 08/31/2020
%% Author: Jack He
%% Servo Dynamics
function [angAccLeft, angAccRight, forceBody, torqueBody] = fcn(torqueLeft, torqueRight, angleLeft, angleRight, omegaLeft, omegaRight, armLength, servoLength, motorLength)
% prop motor mass
m = 0.12;
% prop motor inertia
I = m*motorLength^2;

angAccLeft  = torqueLeft  / I;
angAccRight = torqueRight / I;

centripetalLeft  = m * omegaLeft^2 * motorLength;
centripetalRight = m * omegaRight^2 * motorLength;
tangentialLeft   = m * angAccLeft * motorLength;
tangentialRight  = m * angAccRight * motorLength;

forceAtLeftMotor = [-centripetalLeft*sin(angleLeft);
                                  0;
                    centripetalLeft*cos(angleLeft)];
                 
forceAtRightMotor = [-centripetalRight*sin(angleRight);
                                  0;
                     centripetalRight*cos(angleRight)];


torqueAtLeftServo = [-forceAtLeftMotor(2)*servoLength - forceAtLeftMotor(3)*armLength;
                    forceAtLeftMotor(1)*(servoLength);
                     forceAtLeftMotor(1)*armLength] + [0; torqueLeft; 0];

torqueAtRightServo = [-forceAtRightMotor(2)*servoLength + forceAtRightMotor(3)*armLength;
                    forceAtRightMotor(1)*servoLength;
                    -forceAtRightMotor(1)*armLength] + [0; torqueRight; 0];

forceBody = forceAtLeftMotor + forceAtRightMotor;

torqueBody = torqueAtLeftServo + torqueAtRightServo;

== matlab function multiModeQuad_ROS/Subsystem1/R_EW1 ==
  data: att_sp_NED input; att_sp_Body output; DCM_be input
function att_sp_Body  = fcn(att_sp_NED,DCM_be)
att_sp_Body = [0;0;0];

temp = att_sp_NED(3);


att_sp_Body_temp = deg2rad(DCM_be * att_sp_NED);

att_sp_Body(1) = att_sp_Body_temp(2);
att_sp_Body(2) = -att_sp_Body_temp(1);
att_sp_Body(3) = temp;

== matlab function multiModeQuad_ROS/Subsystem1/Mapping ==
  data: T1 input; T2 input; T3 input; T_B output; tau_B output; T4 input
%% Date created: 08/01/2020
%% Author: Jack He
%% Simulating the dynamics
function [T_B, tau_B] = fcn(T1, T2, T3, T4)

% System input
T_B = [0;
       0;
       -(T1 + T2 + T3 + T4)];

tau_B = [(T3 + T4 - T1 - T2) * 0.15;
         (T2 + T4 - T1 - T3) * 0.15;
         (T2 + T3 - T1 - T4) * 0.20 * 0.2];
